simulink model "Model_Compare"  (R2018a)
settings: Solver=FixedStepDiscrete  StartTime=0.0  StopTime=37  FixedStep=Ts  RelTol=1e-3  EnableMultiTasking=on
values from neighbouring files (symbols this model uses):
  alpha_f0 = states(7)    [IS_2impulse.m]    (also in IS_3impulse.m; IS_4impulse.m; InputShaper.m; InputShaper2.m = 0)
  alpha_r0 = states(8)    [IS_2impulse.m]    (also in IS_3impulse.m; IS_4impulse.m; InputShaper.m; InputShaper2.m = 0)
  Bx_ash_f = 11.7    [ISData.m]    (also in SbWdata.m; pacjeka_params.m)
  Bx_ash_r = 11.1    [ISData.m]    (also in SbWdata.m; pacjeka_params.m)
  Bx_snow_f = 10.2    [ISData.m]    (also in SbWdata.m; pacjeka_params.m)
  Bx_snow_r = 9.71    [ISData.m]    (also in SbWdata.m; pacjeka_params.m)
  Bx_wash_f = 12    [ISData.m]    (also in SbWdata.m; pacjeka_params.m)
  Bx_wash_r = 11.5    [ISData.m]    (also in SbWdata.m; pacjeka_params.m)
  By_ash_f = 8.86    [ISData.m]    (also in SbWdata.m; pacjeka_params.m)
  By_ash_r = 9.30    (= 9.3)    [ISData.m]    (also in SbWdata.m; pacjeka_params.m)
  By_snow_f = 19.1    [ISData.m]    (also in SbWdata.m; pacjeka_params.m)
  By_snow_r = 20.0    (= 20)    [ISData.m]    (also in SbWdata.m; pacjeka_params.m)
  By_wash_f = 10.7    [ISData.m]    (also in SbWdata.m; pacjeka_params.m)
  By_wash_r = 11.3    [ISData.m]    (also in SbWdata.m; pacjeka_params.m)
  Cx_ash_f = 1.69    [ISData.m]    (also in SbWdata.m; pacjeka_params.m)
  Cx_ash_r = 1.69    [ISData.m]    (also in SbWdata.m; pacjeka_params.m)
  Cx_snow_f = 1.96    [ISData.m]    (also in SbWdata.m; pacjeka_params.m)
  Cx_snow_r = 1.96    [ISData.m]    (also in SbWdata.m; pacjeka_params.m)
  Cx_wash_f = 1.80    (= 1.8)    [ISData.m]    (also in SbWdata.m; pacjeka_params.m)
  Cx_wash_r = 1.80    (= 1.8)    [ISData.m]    (also in SbWdata.m; pacjeka_params.m)
  Cy_ash_f = 1.19    [ISData.m]    (also in SbWdata.m; pacjeka_params.m)
  Cy_ash_r = 1.19    [ISData.m]    (also in SbWdata.m; pacjeka_params.m)
  Cy_snow_f = 0.550    (= 0.55)    [ISData.m]    (also in SbWdata.m; pacjeka_params.m)
  Cy_snow_r = 0.550    (= 0.55)    [ISData.m]    (also in SbWdata.m; pacjeka_params.m)
  Cy_wash_f = 1.07    [ISData.m]    (also in SbWdata.m; pacjeka_params.m)
  Cy_wash_r = 1.07    [ISData.m]    (also in SbWdata.m; pacjeka_params.m)
  D_phi = 16000    [ISData.m]    (also in IS_2impulse.m; IS_3impulse.m; IS_4impulse.m; InputShaper.m)
  D_theta = 30960    [ISData.m]    (also in IS_2impulse.m; IS_3impulse.m; IS_4impulse.m; InputShaper.m)
  delta_r = 0    [ISData.m]    (also in IS_2impulse.m; IS_3impulse.m; IS_4impulse.m; InputShaper.m)
  epsilon = 0.4    [ISData.m]    (also in IS_2impulse.m; IS_3impulse.m; IS_4impulse.m; InputShaper.m)
  Ex_ash_f = 0.377    [ISData.m]    (also in SbWdata.m; pacjeka_params.m)
  Ex_ash_r = 0.362    [ISData.m]    (also in SbWdata.m; pacjeka_params.m)
  Ex_snow_f = 0.651    [ISData.m]    (also in SbWdata.m; pacjeka_params.m)
  Ex_snow_r = 0.624    [ISData.m]    (also in SbWdata.m; pacjeka_params.m)
  Ex_wash_f = 0.313    [ISData.m]    (also in SbWdata.m; pacjeka_params.m)
  Ex_wash_r = 0.300    (= 0.3)    [ISData.m]    (also in SbWdata.m; pacjeka_params.m)
  Ey_ash_f = -1.21    [ISData.m]    (also in SbWdata.m; pacjeka_params.m)
  Ey_ash_r = -1.11    [ISData.m]    (also in SbWdata.m; pacjeka_params.m)
  Ey_snow_f = -2.1    [ISData.m]    (also in SbWdata.m; pacjeka_params.m)
  Ey_snow_r = -1.93    [ISData.m]    (also in SbWdata.m; pacjeka_params.m)
  Ey_wash_f = -2.14    [ISData.m]    (also in SbWdata.m; pacjeka_params.m)
  Ey_wash_r = -1.97    [ISData.m]    (also in SbWdata.m; pacjeka_params.m)
  g = 9.81    [ISData.m]    (also in IS_2impulse.m; IS_3impulse.m; IS_4impulse.m; InputShaper.m)
  h = 0.5    [ISData.m]    (also in IS_2impulse.m; IS_3impulse.m; IS_4impulse.m; InputShaper.m)
  Iw = 4    [ISData.m]    (also in IS_2impulse.m; IS_3impulse.m; IS_4impulse.m; InputShaper.m)
  Ixx = 602.1923    [ISData.m]    (also in IS_2impulse.m; IS_3impulse.m; IS_4impulse.m; InputShaper.m)
  Iyy = 2.7370e+03    (= 2737)    [ISData.m]    (also in IS_2impulse.m; IS_3impulse.m; IS_4impulse.m; InputShaper.m)
  Iz = Izz    (= 3070)    [IS_2impulse.m]    (also in IS_3impulse.m; IS_4impulse.m; InputShaper.m; InputShaper2.m)
  Izz = 3070    [ISData.m]    (also in IS_2impulse.m; IS_3impulse.m; IS_4impulse.m; InputShaper.m)
  K_phi = 178000    [ISData.m]    (also in IS_2impulse.m; IS_3impulse.m; IS_4impulse.m; InputShaper.m)
  K_theta = 363540    [ISData.m]    (also in IS_2impulse.m; IS_3impulse.m; IS_4impulse.m; InputShaper.m)
  l = l_f+l_r    (= 2.67)    [IS_2impulse.m]    (also in IS_3impulse.m; IS_4impulse.m; InputShaper.m; InputShaper2.m)
  l_f = 1.2110    (= 1.211)    [ISData.m]    (also in IS_2impulse.m; IS_3impulse.m; IS_4impulse.m; InputShaper.m)
  l_r = 1.4590    (= 1.459)    [ISData.m]    (also in IS_2impulse.m; IS_3impulse.m; IS_4impulse.m; InputShaper.m)
  m = 1830    [ISData.m]    (also in IS_2impulse.m; IS_3impulse.m; IS_4impulse.m; InputShaper.m)
  mu_x_ash_f = 1.20    (= 1.2)    [ISData.m]    (also in SbWdata.m; pacjeka_params.m)
  mu_x_ash_r = 1.20    (= 1.2)    [ISData.m]    (also in SbWdata.m; pacjeka_params.m)
  mu_x_snow_f = 0.407    [ISData.m]    (also in SbWdata.m; pacjeka_params.m)
  mu_x_snow_r = 0.409    [ISData.m]    (also in SbWdata.m; pacjeka_params.m)
  mu_x_wash_f = 1.06    [ISData.m]    (also in SbWdata.m; pacjeka_params.m)
  mu_x_wash_r = 1.07    [ISData.m]    (also in SbWdata.m; pacjeka_params.m)
  mu_y_ash_f = 0.935    [ISData.m]    (also in SbWdata.m; pacjeka_params.m)
  mu_y_ash_r = 0.961    [ISData.m]    (also in SbWdata.m; pacjeka_params.m)
  mu_y_snow_f = 0.383    [ISData.m]    (also in SbWdata.m; pacjeka_params.m)
  mu_y_snow_r = 0.394    [ISData.m]    (also in SbWdata.m; pacjeka_params.m)
  mu_y_wash_f = 0.885    [ISData.m]    (also in SbWdata.m; pacjeka_params.m)
  mu_y_wash_r = 0.911    [ISData.m]    (also in SbWdata.m; pacjeka_params.m)
  omega0 = Vx0/Rw    (= 48.6005830904)    [ISData.m]    (also in IS_2impulse.m = 74.1; IS_3impulse.m = 74.1; IS_4impulse.m = 74.1; InputShaper.m = 55.5666666667)
  omega_f0 = states(5)    [IS_2impulse.m]    (also in IS_3impulse.m; IS_4impulse.m; InputShaper.m; InputShaper2.m = 55.5666666667)
  omega_r0 = states(6)    [IS_2impulse.m]    (also in IS_3impulse.m; IS_4impulse.m; InputShaper.m; InputShaper2.m = 55.5666666667)
  psi0 = states(2)    [IS_2impulse.m]    (also in IS_3impulse.m; IS_4impulse.m; InputShaper.m; InputShaper2.m = 0)
  psi_dot0 = states(1)    [IS_2impulse.m]    (also in IS_3impulse.m; IS_4impulse.m; InputShaper.m; InputShaper2.m = 0)
  Px0 = states(9)    [IS_2impulse.m]    (also in IS_3impulse.m; IS_4impulse.m; InputShaper.m; InputShaper2.m = 0)
  Py0 = states(10)    [IS_2impulse.m]    (also in IS_3impulse.m; IS_4impulse.m; InputShaper.m; InputShaper2.m = 0)
  Re = Rw    (= 0.3)    [IS_2impulse.m]    (also in IS_3impulse.m; IS_4impulse.m; InputShaper.m; InputShaper2.m)
  road = 1    [ISData.m]    (also in IS_2impulse.m; IS_3impulse.m; IS_4impulse.m; InputShaper.m)
  Rw = 0.3430    (= 0.343)    [ISData.m]    (also in IS_2impulse.m = 0.3; IS_3impulse.m = 0.3; IS_4impulse.m = 0.3; InputShaper.m = 0.3)
  sigma = epsilon    (= 0.4)    [IS_2impulse.m]    (also in IS_3impulse.m; IS_4impulse.m; InputShaper.m; InputShaper2.m)
  Ts = 0.001    [ISData.m]    (also in IS_2impulse.m; IS_3impulse.m; IS_4impulse.m; InputShaper.m)
  Tsmall = 0.001    [ISData.m]    (also in IS_2impulse.m; IS_3impulse.m; IS_4impulse.m; InputShaper.m)
  Vx0 = 16.67    [ISData.m]    (also in IS_2impulse.m = states(3); IS_3impulse.m = states(3); IS_4impulse.m = states(3); InputShaper.m = states(3))
  Vy0 = states(4)    [IS_2impulse.m]    (also in IS_3impulse.m; IS_4impulse.m; InputShaper.m; InputShaper2.m = 0)
  w = 0.7700    (= 0.77)    [ISData.m]    (also in IS_2impulse.m; IS_3impulse.m; IS_4impulse.m; InputShaper.m)
undefined symbols (not defined in the file or in its folder): theta_sw_FH
libraries: simulink x2
(part 1 of 3)
settings Model: ExtModeTrigDuration=10000  Creator=srivats  LastModifiedBy=srivats
settings SolverCC: PositivePriorityOrder=on
settings RTWCC: SystemTargetFile=quarc_win64.tlc  TemplateMakefile=quarc_default_tmf  Description=QUARC Win64 Target
settings STFCustomTargetCC: TargetPreCompLibLocation=C:\PROGRA~3\QUARC\lib\2018a\win64\release  TargetLangStandard=C99 (ISO)  ConcurrentExecutionCompliant=on  SystemTargetFile=quarc_win64.tlc
settings GRTTargetCC: TargetPreCompLibLocation=C:\PROGRA~3\QUARC\lib\2018a\win64\release  ParMdlRefBuildCompliant=off  CompOptLevelCompliant=off  CombineOutputUpdateFcns=off  MatFileLogging=off  CPPClassGenCompliant=off  GRTInterface=on  UseToolchainInfoCompliant=off  ExtMode=on  ExtModeMexFile=quarc_comm

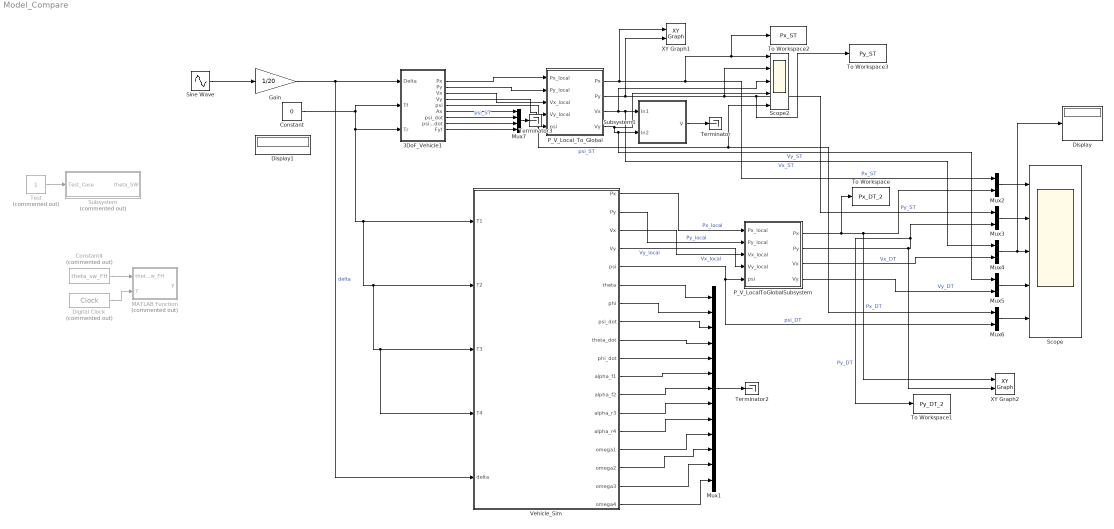
== system Model_Compare ==
  3DoF_Vehicle1 : Subsystem
  Constant : Constant  Value=0
  Constant4 : Constant  Commented=on  Value=theta_sw_FH
  Digital Clock : DigitalClock  Commented=on  SampleTime=0.001
  Display : Display
  Display1 : Display
  Gain : Gain  Gain=1/20
  MATLAB Function : MATLAB Function  Commented=on  TreatAsAtomicUnit=on
  Mux1 : Mux  Inputs=13
  Mux{2..6} (5 alike) : Mux  Inputs=2
  Mux7 : Mux
  P_V_LocalToGlobalSubsystem : Subsystem
  P_V_Local_To_Global : Subsystem
  Scope : Scope  NumInputPorts=5
  Scope2 : Scope  NumInputPorts=5
  Sine Wave : Sin  Amplitude=0.11  Frequency=2*pi/10  SampleTime=0
  Subsystem : Subsystem  Commented=on
  Subsystem1 : Subsystem
  Terminator : Terminator
  Terminator2 : Terminator
  Terminator3 : Terminator
  Test : Constant  Commented=on
  To Workspace : ToWorkspace  VariableName=Px_DT_2  SaveFormat=Timeseries  SampleTime=-1
  To Workspace1 : ToWorkspace  VariableName=Py_DT_2  SaveFormat=Timeseries  SampleTime=-1
  To Workspace2 : ToWorkspace  VariableName=Px_ST  SaveFormat=Timeseries  SampleTime=-1
  To Workspace3 : ToWorkspace  VariableName=Py_ST  SaveFormat=Timeseries  SampleTime=-1
  Vehicle_Sim : Subsystem
  XY Graph1 : simulink/Sinks/XY Graph  xmin=0  xmax=1000  ymin=-100  ymax=100  st=-1
  XY Graph2 : simulink/Sinks/XY Graph  xmin=0  xmax=1000  ymin=-100  ymax=100  st=-1
  wires:
  3DoF_Vehicle1/7(psi_dot) -> Mux7/2  "psi_ST"
  Subsystem1/1(V) -> Terminator/1
  3DoF_Vehicle1/3(Vx) -> P_V_Local_To_Global/3(Vx_local)
  3DoF_Vehicle1/1(Px) -> P_V_Local_To_Global/1(Px_local)
  3DoF_Vehicle1/4(Vy) -> P_V_Local_To_Global/4(Vy_local)
  3DoF_Vehicle1/2(Py) -> P_V_Local_To_Global/2(Py_local)
  P_V_Local_To_Global/4(Vy) -> Scope2/4, Mux5/1, Subsystem1/2(In2)  "Vy_ST"
  P_V_Local_To_Global/3(Vx) -> Scope2/3, Mux4/1, Subsystem1/1(In1)  "Vx_ST"
  Gain/1 -> Vehicle_Sim/5("delta "), 3DoF_Vehicle1/1(Delta)  "delta"
  P_V_LocalToGlobalSubsystem/4(Vy) -> Mux5/2  "Vy_DT"
  Vehicle_Sim/6(theta) -> Mux1/1
  Vehicle_Sim/7(phi) -> Mux1/2
  Vehicle_Sim/17(omega3) -> Mux1/12
  Vehicle_Sim/2(Py) -> P_V_LocalToGlobalSubsystem/2(Py_local)  "Py_local"
  Vehicle_Sim/18(omega4) -> Mux1/13
  Vehicle_Sim/11(alpha_f1) -> Mux1/6
  P_V_LocalToGlobalSubsystem/2(Py) -> XY Graph2/2, To Workspace1/1, Mux3/2  "Py_DT"
  P_V_LocalToGlobalSubsystem/3(Vx) -> Mux4/2  "Vx_DT"
  P_V_LocalToGlobalSubsystem/1(Px) -> To Workspace/1, XY Graph2/1, Mux2/2  "Px_DT"
  Vehicle_Sim/8(psi_dot) -> Mux1/3
  Vehicle_Sim/4(Vy) -> P_V_LocalToGlobalSubsystem/4(Vy_local)  "Vy_local"
  Mux1/1 -> Terminator2/1
  Vehicle_Sim/1(Px) -> P_V_LocalToGlobalSubsystem/1(Px_local)  "Px_local"
  Vehicle_Sim/12(alpha_f2) -> Mux1/7
  Vehicle_Sim/10(phi_dot) -> Mux1/5
  Vehicle_Sim/3(Vx) -> P_V_LocalToGlobalSubsystem/3(Vx_local)  "Vx_local"
  Vehicle_Sim/14(alpha_r4) -> Mux1/9
  Vehicle_Sim/15(omega1) -> Mux1/10
  Vehicle_Sim/5(psi) -> Mux6/2, P_V_LocalToGlobalSubsystem/5(psi)  "psi_DT"
  Vehicle_Sim/16(omega2) -> Mux1/11
  Vehicle_Sim/9(theta_dot) -> Mux1/4
  Vehicle_Sim/13(alpha_r3) -> Mux1/8
  P_V_Local_To_Global/1(Px) -> XY Graph1/1, To Workspace2/1, Scope2/1, Mux2/1  "Px_ST"
  Mux2/1 -> Scope/1
  P_V_Local_To_Global/2(Py) -> XY Graph1/2, Scope2/2, To Workspace3/1, Mux3/1  "Py_ST"
  Mux3/1 -> Scope/2
  Mux4/1 -> Display/1, Scope/3
  Mux5/1 -> Scope/4
  Mux6/1 -> Scope/5
  Constant/1 -> Vehicle_Sim/4(T4), Vehicle_Sim/3(T3), Vehicle_Sim/2(T2), Vehicle_Sim/1(T1), 3DoF_Vehicle1/3(Tr), 3DoF_Vehicle1/2(Tf)
  3DoF_Vehicle1/6(Ax) -> Mux7/1
  3DoF_Vehicle1/8(psi_ddot) -> Mux7/3
  3DoF_Vehicle1/9(Fyf) -> Mux7/4
  Mux7/1 -> Terminator3/1
  3DoF_Vehicle1/5(psi) -> Scope2/5, Mux6/1, P_V_Local_To_Global/5(psi)  "psi_ST"
  Test/1 -> Subsystem/1(Test_Case)
  Digital Clock/1 -> MATLAB Function/2(T)
  Constant4/1 -> MATLAB Function/1(theta_sw_FH)
  Sine Wave/1 -> Gain/1

== system Model_Compare/3DoF_Vehicle1 ==
  Delta : Inport
  Tf : Inport  Port=2
  Tr : Inport  Port=3
  Add : Sum
  Add1 : Sum
  Add2 : Sum
  Constant : Constant  Value=Px0
  Constant1 : Constant  Value=Py0
  Constant2 : Constant  Value=psi0
  Constant3 : Constant  Value=psi_dot0
  Constant4 : Constant  Value=Vy0
  Constant5 : Constant  Value=Vx0
  Constant6 : Constant  Value=omega_f0
  Constant7 : Constant  Value=omega_r0
  Constant8 : Constant  Value=alpha_f0
  Constant9 : Constant  Value=alpha_r0
  Delay : Delay  DelayLength=1  InitialConditionSource=Input port  SampleTime=Tsmall
      settings: InputPortMap=u0,p4
  Delay1 : Delay  DelayLength=1  InitialConditionSource=Input port  SampleTime=Tsmall
      settings: InputPortMap=u0,p4
  Demux : Demux  Outputs=8
  Demux1 : Demux  Outputs=2
  Gain : Gain  Gain=Tsmall
  Gain1 : Gain  Gain=Tsmall
  Gain2 : Gain  Gain=Tsmall
  Mux : Mux  Inputs=8
  Mux1 : Mux  Inputs=2
  Mux2 : Mux  Inputs=2
  Mux3 : Mux  Inputs=8
  Subsystem1 : Subsystem
  Px : Outport
  Py : Outport  Port=2
  Vx : Outport  Port=3
  Vy : Outport  Port=4
  psi : Outport  Port=5
  Ax : Outport  Port=6
  psi_dot : Outport  Port=7
  psi_ddot : Outport  Port=8
  Fyf : Outport  Port=9
  wires:
  Demux/1 -> psi/1, Add/2  "psi_curr"
  Delay/1 -> Demux/1
  Demux/6 -> Subsystem1/6(omega_r_curr)  "omega_r_curr"
  Gain/1 -> Add/1
  Delta/1 -> Subsystem1/1(Delta)
  Subsystem1/4(omega_f_next) -> Mux/5  "omega_f_next"
  Subsystem1/1(psi_dot_next) -> Mux/2, Gain/1  "psi_dot_next"
  Add/1 -> Mux/1  "psi_next"
  Tr/1 -> Subsystem1/8(Tr)
  Tf/1 -> Subsystem1/7(Tf)
  Subsystem1/3(Vx_next) -> Mux/4  "Vx_next"
  Demux/2 -> psi_dot/1, Subsystem1/2(psi_dot_curr)  "psi_dot_curr"
  Mux/1 -> Delay/1
  Demux/4 -> Vx/1, Gain1/1, Subsystem1/3(Vx_curr)  "Vx_curr"
  Demux/3 -> Gain2/1, Subsystem1/4(Vy_curr), Vy/1  "Vy_curr"
  Demux/5 -> Subsystem1/5(omega_f_curr)  "omega_f_curr"
  Subsystem1/2(Vy_next) -> Mux/3  "Vy_next"
  Subsystem1/5(omega_r_next) -> Mux/6  "omega_r_next"
  Gain1/1 -> Add1/1
  Gain2/1 -> Add2/1
  Mux1/1 -> Delay1/1
  Add1/1 -> Mux1/1  "Px_next"
  Add2/1 -> Mux1/2  "Py_next"
  Mux2/1 -> Delay1/2
  Constant/1 -> Mux2/1
  Constant1/1 -> Mux2/2
  Delay1/1 -> Demux1/1
  Demux1/1 -> Add1/2, Px/1  "Px_curr"
  Demux1/2 -> Add2/2, Py/1  "Py_curr"
  Constant7/1 -> Mux3/6
  Constant6/1 -> Mux3/5
  Constant3/1 -> Mux3/2
  Constant5/1 -> Mux3/4
  Constant4/1 -> Mux3/3
  Constant2/1 -> Mux3/1
  Mux3/1 -> Delay/2
  Subsystem1/6(alpha_f_next) -> Mux/7  "alpha_f_next"
  Subsystem1/7(alpha_r_next) -> Mux/8  "alpha_r_next"
  Constant8/1 -> Mux3/7
  Constant9/1 -> Mux3/8
  Demux/7 -> Subsystem1/9(alpha_f_curr)  "alpha_f_curr"
  Demux/8 -> Subsystem1/10(alpha_r_curr)  "alpha_r_curr"
  Subsystem1/8(Ax) -> Ax/1
  Subsystem1/9(psi_ddot) -> psi_ddot/1
  Subsystem1/10(Fyf) -> Fyf/1

== system Model_Compare/P_V_LocalToGlobalSubsystem ==
  Px_local : Inport  OutDataTypeStr=double  SampleTime=Ts
  Py_local : Inport  Port=2  OutDataTypeStr=double  SampleTime=Ts
  Vx_local : Inport  Port=3  OutDataTypeStr=double  SampleTime=Ts
  Vy_local : Inport  Port=4  OutDataTypeStr=double  SampleTime=Ts
  psi : Inport  Port=5  OutDataTypeStr=double  SampleTime=Ts
  Add : Sum  Inputs=+-
  Add1 : Sum
  Add2 : Sum  Inputs=+-
  Add3 : Sum
  Cos : Trigonometry  Operator=cos
  Product{,1..7} (8 alike) : Product
  Sin : Trigonometry
  Px : Outport  OutDataTypeStr=double  SampleTime=Ts
  Py : Outport  Port=2  OutDataTypeStr=double  SampleTime=Ts
  Vx : Outport  Port=3  OutDataTypeStr=double  SampleTime=Ts
  Vy : Outport  Port=4  OutDataTypeStr=double  SampleTime=Ts
  wires:
  Px_local/1 -> Product6/1, Product4/1  "Px_local"
  Py_local/1 -> Product7/1, Product5/1  "Py_local"
  Vx_local/1 -> Product2/1, Product/2  "Vx_local"
  Product5/1 -> Add2/2
  Product4/1 -> Add2/1
  Add2/1 -> Px/1  "Px"
  Product7/1 -> Add3/2
  Vy_local/1 -> Product3/1, Product1/2  "Vy_local"
  psi/1 -> Sin/1, Cos/1  "psi"
  Cos/1 -> Product3/2, Product/1, Product7/2, Product4/2  "cosPsi"
  Add3/1 -> Py/1  "Py"
  Product2/1 -> Add1/1
  Product1/1 -> Add/2
  Add/1 -> Vx/1  "Vx"
  Add1/1 -> Vy/1  "Vy"
  Product6/1 -> Add3/1
  Product3/1 -> Add1/2
  Product/1 -> Add/1
  Sin/1 -> Product2/2, Product1/1, Product6/2, Product5/2  "sinPsi"

== system Model_Compare/P_V_Local_To_Global ==
  Px_local : Inport  OutDataTypeStr=double  SampleTime=Ts
  Py_local : Inport  Port=2  OutDataTypeStr=double  SampleTime=Ts
  Vx_local : Inport  Port=3  OutDataTypeStr=double  SampleTime=Ts
  Vy_local : Inport  Port=4  OutDataTypeStr=double  SampleTime=Ts
  psi : Inport  Port=5  OutDataTypeStr=double  SampleTime=Ts
  Add : Sum  Inputs=+-
  Add1 : Sum
  Add2 : Sum  Inputs=+-
  Add3 : Sum
  Cos : Trigonometry  Operator=cos
  Product{,1..7} (8 alike) : Product
  Sin : Trigonometry
  Px : Outport  OutDataTypeStr=double  SampleTime=Ts
  Py : Outport  Port=2  OutDataTypeStr=double  SampleTime=Ts
  Vx : Outport  Port=3  OutDataTypeStr=double  SampleTime=Ts
  Vy : Outport  Port=4  OutDataTypeStr=double  SampleTime=Ts
  wires:
  Px_local/1 -> Product4/1, Product6/2
  Py_local/1 -> Product7/1, Product5/1
  Vx_local/1 -> Product3/1, Product/1
  Product5/1 -> Add2/2
  Product4/1 -> Add2/1
  Add2/1 -> Px/1  "Px"
  Product7/1 -> Add3/2
  Sin/1 -> Product6/1, Product5/2, Product3/2, Product1/1  "sinPsi"
  Vy_local/1 -> Product1/2, Product2/2
  psi/1 -> Sin/1, Cos/1
  Cos/1 -> Product7/2, Product4/2, Product2/1, Product/2  "cosPsi"
  Add3/1 -> Py/1  "Py"
  Product2/1 -> Add1/1
  Product1/1 -> Add/2
  Add/1 -> Vx/1  "Vx"
  Add1/1 -> Vy/1  "Vy"
  Product6/1 -> Add3/1
  Product3/1 -> Add1/2
  Product/1 -> Add/1

== system Model_Compare/Subsystem ==
  Test_Case : Inport
  If : If  IfExpression=u1==1  ElseIfExpressions=u1==2  ShowElse=off
  If Action Subsystem : Subsystem  TreatAsAtomicUnit=on
  If Action Subsystem1 : Subsystem  TreatAsAtomicUnit=on
  Merge : Merge
  theta_SW : Outport
  wires:
  Merge/1 -> theta_SW/1
  Test_Case/1 -> If/1
  If Action Subsystem/1(Out1) -> Merge/1
  If/1 -> If Action Subsystem/Action
  If/2 -> If Action Subsystem1/Action
  If Action Subsystem1/1(Out1) -> Merge/2

== system Model_Compare/Subsystem1 ==
  In1 : Inport
  In2 : Inport  Port=2
  Add : Sum
  Sqrt : Sqrt  SaturateOnIntegerOverflow=on
  Square : Math  Operator=square  SaturateOnIntegerOverflow=on
  Square1 : Math  Operator=square  SaturateOnIntegerOverflow=on
  V : Outport
  wires:
  Square1/1 -> Add/2
  In1/1 -> Square/1
  Add/1 -> Sqrt/1
  Square/1 -> Add/1
  Sqrt/1 -> V/1  "V"
  In2/1 -> Square1/1

== system Model_Compare/Vehicle_Sim ==
  T1 : Inport  OutDataTypeStr=double  SampleTime=Ts
  T2 : Inport  Port=2  OutDataTypeStr=double  SampleTime=Ts
  T3 : Inport  Port=3  OutDataTypeStr=double  SampleTime=Ts
  T4 : Inport  Port=4  OutDataTypeStr=double  SampleTime=Ts
  "delta " : Inport  Port=5
  Add1 : Sum
  Add2 : Sum
  Delay2 : Delay  DelayLength=1  SampleTime=Tsmall
  Delay3 : Delay  DelayLength=1  SampleTime=Tsmall
  Demux : Demux  Outputs=11
  Demux1 : Demux
  Gain1 : Gain  Gain=Tsmall
  Gain2 : Gain  Gain=Tsmall
  Mux : Mux  Inputs=11
      settings: DisplayOption=signals
  Mux1 : Mux
      settings: DisplayOption=signals
  Vehicle_model : Subsystem
  Vx_delay : Delay  DelayLength=1  InitialCondition=Vx0  SampleTime=Tsmall
  omega_delay : Delay  DelayLength=1  InitialCondition=omega0*ones(4,1)  SampleTime=Tsmall
  otherstates_delay : Delay  DelayLength=1  InitialCondition=zeros(11,1)  SampleTime=Tsmall
  Px : Outport  OutDataTypeStr=double  SampleTime=Tsmall
  Py : Outport  Port=2  OutDataTypeStr=double  SampleTime=Tsmall
  Vx : Outport  Port=3  OutDataTypeStr=double  SampleTime=Tsmall
  Vy : Outport  Port=4  OutDataTypeStr=double  SampleTime=Tsmall
  psi : Outport  Port=5  OutDataTypeStr=double  SampleTime=Tsmall
  theta : Outport  Port=6  OutDataTypeStr=double  SampleTime=Tsmall
  phi : Outport  Port=7  OutDataTypeStr=double  SampleTime=Tsmall
  psi_dot : Outport  Port=8  OutDataTypeStr=double  SampleTime=Tsmall
  theta_dot : Outport  Port=9  OutDataTypeStr=double  SampleTime=Tsmall
  phi_dot : Outport  Port=10  OutDataTypeStr=double  SampleTime=Tsmall
  alpha_f1 : Outport  Port=11  OutDataTypeStr=double  SampleTime=Tsmall
  alpha_f2 : Outport  Port=12  OutDataTypeStr=double  SampleTime=Tsmall
  alpha_r3 : Outport  Port=13  OutDataTypeStr=double  SampleTime=Tsmall
  alpha_r4 : Outport  Port=14  OutDataTypeStr=double  SampleTime=Tsmall
  omega1 : Outport  Port=15  OutDataTypeStr=double  SampleTime=Tsmall
  omega2 : Outport  Port=16  OutDataTypeStr=double  SampleTime=Tsmall
  omega3 : Outport  Port=17  OutDataTypeStr=double  SampleTime=Tsmall
  omega4 : Outport  Port=18  OutDataTypeStr=double  SampleTime=Tsmall
  wires:
  Vehicle_model/14(theta_next) -> Mux/9  "theta_next"
  Vehicle_model/12(psi_next) -> Mux/7  "psi_next"
  Vehicle_model/11(psi_dot_next) -> Mux/6  "psi_dot_next"
  Vehicle_model/15(phi_dot_next) -> Mux/10  "phi_dot_next"
  Mux/1 -> otherstates_delay/1
  Vehicle_model/3(alpha_f1_next) -> Mux/2  "alpha_f1_next"
  Vehicle_model/5(alpha_r3_next) -> Mux/4  "alpha_r3_next"
  Vehicle_model/9(omega3_next) -> Mux1/3  "omega3_next"
  Vehicle_model/8(omega2_next) -> Mux1/2  "omega2_next"
  Vehicle_model/13(theta_dot_next) -> Mux/8  "theta_dot_next"
  Vehicle_model/4(alpha_f2_next) -> Mux/3  "alpha_f2_next"
  Vehicle_model/6(alpha_r4_next) -> Mux/5  "alpha_r4_next"
  Vehicle_model/10(omega4_next) -> Mux1/4  "omega4_next"
  Vehicle_model/1(Vx_next) -> Vx_delay/1  "Vx_next"
  Demux/1 -> Gain2/1, Vy/1, Vehicle_model/6(Vy_curr)
  Vehicle_model/7(omega1_next) -> Mux1/1  "omega1_next"
  Demux1/3 -> omega3/1, Vehicle_model/13(omega3_curr)
  Demux/5 -> Vehicle_model/10(alpha_r4_curr), alpha_r4/1
  Demux/8 -> theta_dot/1, Vehicle_model/17(theta_dot_curr)
  Vehicle_model/16(phi_next) -> Mux/11  "phi_next"
  Vehicle_model/2(Vy_next) -> Mux/1  "Vy_next"
  T1/1 -> Vehicle_model/1(T1)
  Add2/1 -> Delay3/1
  Delay3/1 -> Py/1, Add2/2  "Py_curr"
  Add1/1 -> Delay2/1  "Px_next"
  Delay2/1 -> Px/1, Add1/2  "Px_curr"
  Gain1/1 -> Add1/1
  Gain2/1 -> Add2/1
  T3/1 -> Vehicle_model/3(T3)
  T4/1 -> Vehicle_model/4(T4)
  T2/1 -> Vehicle_model/2(T2)
  otherstates_delay/1 -> Demux/1
  Demux/4 -> Vehicle_model/9(alpha_r3_curr), alpha_r3/1
  Demux/11 -> phi/1, Vehicle_model/19(phi_curr)
  Demux/2 -> Vehicle_model/7(alpha_f1_curr), alpha_f1/1
  Demux/3 -> Vehicle_model/8(alpha_f2_curr), alpha_f2/1
  Demux1/4 -> omega4/1, Vehicle_model/14(omega4_curr)
  Demux/7 -> psi/1, Vehicle_model/16(psi_curr)
  Demux/9 -> theta/1, Vehicle_model/18(theta_curr)
  Demux/10 -> phi_dot/1, Vehicle_model/20(phi_dot_curr)
  Demux/6 -> psi_dot/1, Vehicle_model/15(psi_dot_curr)
  Demux1/2 -> omega2/1, Vehicle_model/12(omega2_curr)
  Vx_delay/1 -> Vx/1, Vehicle_model/5(Vx_curr), Gain1/1
  Demux1/1 -> omega1/1, Vehicle_model/11(omega1_curr)
  Mux1/1 -> omega_delay/1
  omega_delay/1 -> Demux1/1
  "delta "/1 -> Vehicle_model/21(delta)

== system Model_Compare/3DoF_Vehicle1/Subsystem1 ==
  Delta : Inport
  psi_dot_curr : Inport  Port=2
  Vx_curr : Inport  Port=3
  Vy_curr : Inport  Port=4
  omega_f_curr : Inport  Port=5
  omega_r_curr : Inport  Port=6
  Tf : Inport  Port=7
  Tr : Inport  Port=8
  alpha_f_curr : Inport  Port=9
  alpha_r_curr : Inport  Port=10
  Cos : Trigonometry  Operator=cos
  Demux1 : Demux  Outputs=8
  Demux2 : Demux  Outputs=8
  Fx_Fy_Subsystem : Subsystem
  Fz_Subsystem : Subsystem
  Omega_k_alpha_Subsystem : Subsystem
  Pacjeka_parameters_Subsystem : Subsystem
  Psi_ddot_subsystem : Subsystem
  Sin : Trigonometry
  Vxdot_subsystem : Subsystem
  Vydot_subsystem : Subsystem
  surface : Constant  Value=road
  psi_dot_next : Outport
  Vy_next : Outport  Port=2
  Vx_next : Outport  Port=3
  omega_f_next : Outport  Port=4
  omega_r_next : Outport  Port=5
  alpha_f_next : Outport  Port=6
  alpha_r_next : Outport  Port=7
  Ax : Outport  Port=8
  psi_ddot : Outport  Port=9
  Fyf : Outport  Port=10
  wires:
  Omega_k_alpha_Subsystem/4(k_r) -> Fx_Fy_Subsystem/21(k_r)
  Fx_Fy_Subsystem/2(Fx_r) -> Vxdot_subsystem/4(Fxr), Omega_k_alpha_Subsystem/10(Fx_r)
  Fx_Fy_Subsystem/1(Fx_f) -> Omega_k_alpha_Subsystem/9(Fx_f), Vxdot_subsystem/3(Fxf), Psi_ddot_subsystem/5(Fxf), Vydot_subsystem/5(Fxf)
  Omega_k_alpha_Subsystem/3(k_f) -> Fx_Fy_Subsystem/22(k_f)
  Sin/1 -> Fx_Fy_Subsystem/24(sinDelta), Vxdot_subsystem/7(sinDelta), Vydot_subsystem/7(sinDelta), Psi_ddot_subsystem/2(sinDelta)
  Vydot_subsystem/1(Vy_next) -> Vy_next/1
  Fx_Fy_Subsystem/3(Fy_f) -> Fyf/1, Psi_ddot_subsystem/3(Fyf), Vydot_subsystem/3(Fyf), Vxdot_subsystem/5(Fyf)
  psi_dot_curr/1 -> Omega_k_alpha_Subsystem/6(psi_dot), Vydot_subsystem/1(psi_dot_curr), Vxdot_subsystem/1(psi_dot_curr), Psi_ddot_subsystem/6(psi_dot_curr)
  Fx_Fy_Subsystem/4(Fy_r) -> Psi_ddot_subsystem/4(Fyr), Vydot_subsystem/4(Fyr)
  Cos/1 -> Fx_Fy_Subsystem/23(cosDelta), Vxdot_subsystem/6(cosDelta), Vydot_subsystem/6(cosDelta), Psi_ddot_subsystem/1(cosDelta)
  Tf/1 -> Omega_k_alpha_Subsystem/7(Tf)
  Demux1/7 -> Fx_Fy_Subsystem/17(E_x_f)  "E_x_f"
  omega_f_curr/1 -> Omega_k_alpha_Subsystem/4(omega_f_curr)
  Vy_curr/1 -> Omega_k_alpha_Subsystem/3(Vy), Vxdot_subsystem/2(Vy_curr), Vydot_subsystem/8(Vy_curr)
  Pacjeka_parameters_Subsystem/1(front) -> Demux1/1
  Omega_k_alpha_Subsystem/6(omega_r_next) -> omega_r_next/1
  Delta/1 -> Omega_k_alpha_Subsystem/1(delta), Sin/1, Cos/1
  Vx_curr/1 -> Omega_k_alpha_Subsystem/2(Vx), Vydot_subsystem/2(Vx_curr), Vxdot_subsystem/8(Vx_curr)
  Demux1/1 -> Fx_Fy_Subsystem/11(mu_x_f)  "mu_x_f"
  Vxdot_subsystem/1(Vx_next) -> Vx_next/1
  Omega_k_alpha_Subsystem/5(omega_f_next) -> omega_f_next/1
  Demux2/4 -> Fx_Fy_Subsystem/6(C_y_r)  "C_y_r"
  Fz_Subsystem/1(Fz_f) -> Fx_Fy_Subsystem/1(Fz_f)
  Tr/1 -> Omega_k_alpha_Subsystem/8(Tr)
  omega_r_curr/1 -> Omega_k_alpha_Subsystem/5(omega_r_curr)
  surface/1 -> Pacjeka_parameters_Subsystem/1(surface_condition)
  Pacjeka_parameters_Subsystem/2(rear) -> Demux2/1
  Demux2/7 -> Fx_Fy_Subsystem/9(E_x_r)  "E_x_r"
  Fz_Subsystem/2(Fz_r) -> Fx_Fy_Subsystem/2(Fz_r)
  Demux1/6 -> Fx_Fy_Subsystem/16(B_y_f)  "B_y_f"
  Demux2/6 -> Fx_Fy_Subsystem/8(B_y_r)  "B_y_r"
  Demux2/2 -> Fx_Fy_Subsystem/4(mu_y_r)  "mu_y_r"
  Demux1/8 -> Fx_Fy_Subsystem/18(E_y_f)  "E_y_f"
  Demux2/5 -> Fx_Fy_Subsystem/7(B_x_r)  "B_x_r"
  Psi_ddot_subsystem/1(psi_dot_next) -> psi_dot_next/1
  Demux2/8 -> Fx_Fy_Subsystem/10(E_y_r)  "E_y_r"
  Demux2/1 -> Fx_Fy_Subsystem/3(mu_x_r)  "mu_x_r"
  Demux1/3 -> Fx_Fy_Subsystem/13(C_x_f)  "C_x_f"
  Demux1/4 -> Fx_Fy_Subsystem/14(C_y_f)  "C_y_f"
  Demux1/2 -> Fx_Fy_Subsystem/12(mu_y_f)  "mu_y_f"
  Demux1/5 -> Fx_Fy_Subsystem/15(B_x_f)  "B_x_f"
  Demux2/3 -> Fx_Fy_Subsystem/5(C_x_r)  "C_x_r"
  Omega_k_alpha_Subsystem/1(alpha_f_next) -> alpha_f_next/1
  Omega_k_alpha_Subsystem/2(alpha_r_next) -> alpha_r_next/1
  alpha_r_curr/1 -> Fx_Fy_Subsystem/20(alpha_r), Omega_k_alpha_Subsystem/12(alpha_r_curr)
  alpha_f_curr/1 -> Fx_Fy_Subsystem/19(alpha_f), Omega_k_alpha_Subsystem/11(alpha_f_curr)
  Vxdot_subsystem/2(Ax) -> Ax/1
  Psi_ddot_subsystem/2(psi_ddot) -> psi_ddot/1

== system Model_Compare/Subsystem/If Action Subsystem ==
  Action Port : ActionPort  ActionType=then
  From Workspace : FromWorkspace  VariableName=theta_SW_FH  SampleTime=0
  Out1 : Outport
  wires:
  From Workspace/1 -> Out1/1

== system Model_Compare/Subsystem/If Action Subsystem1 ==
  Action Port : ActionPort  ActionType=elseif
  Constant : Constant  Value=0
  Out1 : Outport
  wires:
  Constant/1 -> Out1/1

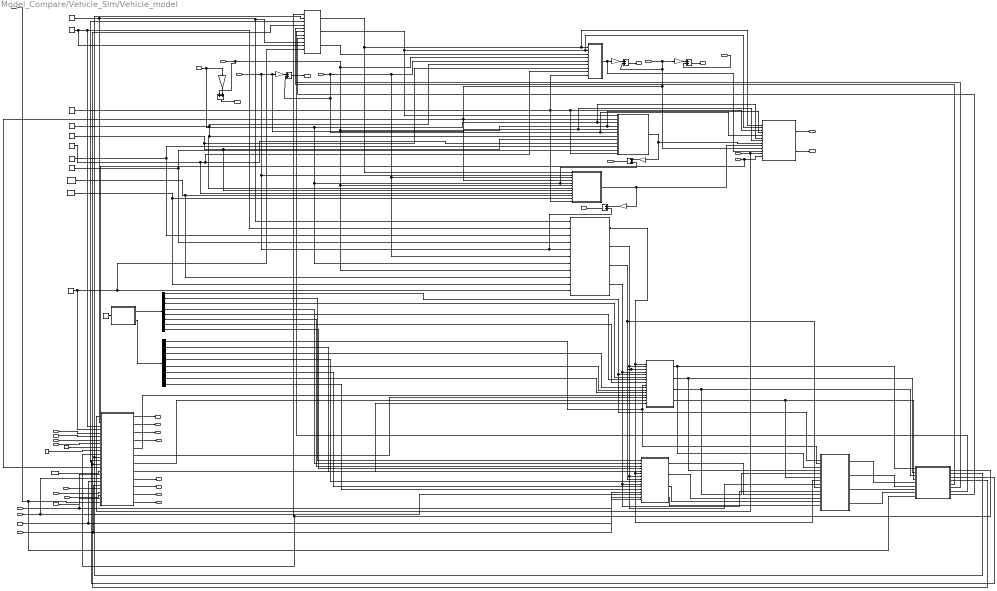
== system Model_Compare/Vehicle_Sim/Vehicle_model ==
  T1 : Inport  OutDataTypeStr=double  SampleTime=Ts
  T2 : Inport  Port=2  OutDataTypeStr=double  SampleTime=Ts
  T3 : Inport  Port=3  OutDataTypeStr=double  SampleTime=Ts
  T4 : Inport  Port=4  OutDataTypeStr=double  SampleTime=Ts
  Vx_curr : Inport  Port=5  OutDataTypeStr=double  SampleTime=Tsmall
  Vy_curr : Inport  Port=6  OutDataTypeStr=double  SampleTime=Tsmall
  alpha_f1_curr : Inport  Port=7  OutDataTypeStr=double  SampleTime=Tsmall
  alpha_f2_curr : Inport  Port=8  OutDataTypeStr=double  SampleTime=Tsmall
  alpha_r3_curr : Inport  Port=9  OutDataTypeStr=double  SampleTime=Tsmall
  alpha_r4_curr : Inport  Port=10  OutDataTypeStr=double  SampleTime=Tsmall
  omega1_curr : Inport  Port=11  OutDataTypeStr=double  SampleTime=Tsmall
  omega2_curr : Inport  Port=12  OutDataTypeStr=double  SampleTime=Tsmall
  omega3_curr : Inport  Port=13  OutDataTypeStr=double  SampleTime=Tsmall
  omega4_curr : Inport  Port=14  OutDataTypeStr=double  SampleTime=Tsmall
  psi_dot_curr : Inport  Port=15  OutDataTypeStr=double  SampleTime=Tsmall
  psi_curr : Inport  Port=16  OutDataTypeStr=double  SampleTime=Tsmall
  theta_dot_curr : Inport  Port=17  OutDataTypeStr=double  SampleTime=Tsmall
  theta_curr : Inport  Port=18  OutDataTypeStr=double  SampleTime=Tsmall
  phi_curr : Inport  Port=19  OutDataTypeStr=double  SampleTime=Tsmall
  phi_dot_curr : Inport  Port=20  OutDataTypeStr=double  SampleTime=Tsmall
  delta : Inport  Port=21  OutDataTypeStr=double  SampleTime=Tsmall
  Add{,1..5} (6 alike) : Sum
  D_phi : Constant  Value=D_phi
  D_theta : Constant  Value=D_theta
  Demux1 : Demux  Outputs=8
  Demux2 : Demux  Outputs=8
  F_M_subsystem : Subsystem
  Fx0_Subsystem : Subsystem
  Fy0_Subsystem : Subsystem
  Fy0_to_Fy_subsystem : Subsystem
  Fz_Subsystem : Subsystem
  Gain{,1..5} (6 alike) : Gain  Gain=Tsmall
  Iw : Constant  Value=Iw
  Ixx : Constant  Value=Ixx
  Iyy : Constant  Value=Iyy
  Izz : Constant  Value=Izz
  K_phi : Constant  Value=K_phi
  K_theta : Constant  Value=K_theta
  Pacjeka_parameters_Subsystem : Subsystem
  Rw : Constant  Value=Rw
  Vx_Vy_Subsystem : Subsystem
  epsilon : Constant  Value=epsilon
  h : Constant  Value=h
  l_f : Constant  Value=l_f
  l_r : Constant  Value=l_r
  local_to_global_Fx_Fy_Subsystem : Subsystem
  omega_alpha_and_k_values_subsystem : Subsystem
  phi_subsystem : Subsystem
  psi_subsystem : Subsystem
  surface : Constant  Value=road
  theta_subsystem : Subsystem
  w : Constant  Value=w
  Vx_next : Outport  OutDataTypeStr=double  SampleTime=Tsmall
  Vy_next : Outport  Port=2  OutDataTypeStr=double  SampleTime=Tsmall
  alpha_f1_next : Outport  Port=3  OutDataTypeStr=double  SampleTime=Tsmall
  alpha_f2_next : Outport  Port=4  OutDataTypeStr=double  SampleTime=Tsmall
  alpha_r3_next : Outport  Port=5  OutDataTypeStr=double  SampleTime=Tsmall
  alpha_r4_next : Outport  Port=6  OutDataTypeStr=double  SampleTime=Tsmall
  omega1_next : Outport  Port=7  OutDataTypeStr=double  SampleTime=Tsmall
  omega2_next : Outport  Port=8  OutDataTypeStr=double  SampleTime=Tsmall
  omega3_next : Outport  Port=9  OutDataTypeStr=double  SampleTime=Tsmall
  omega4_next : Outport  Port=10  OutDataTypeStr=double  SampleTime=Tsmall
  psi_dot_next : Outport  Port=11  OutDataTypeStr=double  SampleTime=Tsmall
  psi_next : Outport  Port=12  OutDataTypeStr=double  SampleTime=Tsmall
  theta_dot_next : Outport  Port=13  OutDataTypeStr=double  SampleTime=Tsmall
  theta_next : Outport  Port=14  OutDataTypeStr=double  SampleTime=Tsmall
  phi_dot_next : Outport  Port=15  OutDataTypeStr=double  SampleTime=Tsmall
  phi_next : Outport  Port=16  OutDataTypeStr=double  SampleTime=Tsmall
  wires:
  Add/1 -> psi_dot_next/1
  Gain4/1 -> Add4/1
  Gain5/1 -> Add5/2
  Add4/1 -> phi_dot_next/1
  Add5/1 -> phi_next/1
  omega1_curr/1 -> omega_alpha_and_k_values_subsystem/22(omega1_curr)
  omega3_curr/1 -> omega_alpha_and_k_values_subsystem/24(omega3_curr)
  omega_alpha_and_k_values_subsystem/11(omega3_next) -> omega3_next/1
  omega_alpha_and_k_values_subsystem/12(omega4_next) -> omega4_next/1
  F_M_subsystem/2(FY) -> phi_subsystem/1(FY), Vx_Vy_Subsystem/2(FY), psi_subsystem/2(FY)  "Fy"
  theta_curr/1 -> Add3/2, Vx_Vy_Subsystem/5(theta), phi_subsystem/6(theta), psi_subsystem/5(theta), Fz_Subsystem/6(theta), theta_subsystem/3(theta)
  Ixx/1 -> psi_subsystem/6(Ixx), theta_subsystem/7(Ixx), phi_subsystem/7(Ixx)  "Ixx"
  phi_dot_curr/1 -> Vx_Vy_Subsystem/6(phi_dot), phi_subsystem/3(phi_dot), Add4/2, theta_subsystem/5(phi_dot), Fz_Subsystem/7(phi_dot), Gain5/1  "phi_dot"
  Izz/1 -> theta_subsystem/9(Izz), psi_subsystem/8(Izz), phi_subsystem/9(Izz)  "Izz"
  theta_subsystem/1(theta_ddot) -> Vx_Vy_Subsystem/9(theta_ddot), Gain2/1  "theta_ddot"
  K_phi/1 -> Fz_Subsystem/3(k_phi), phi_subsystem/10(K_phi)  "k_phi"
  F_M_subsystem/1(FX) -> theta_subsystem/1(FX), Vx_Vy_Subsystem/1(FX), psi_subsystem/1(FX)  "Fx"
  phi_curr/1 -> Add5/1, Fz_Subsystem/8(phi), theta_subsystem/6(phi), Vx_Vy_Subsystem/4(phi), phi_subsystem/4(phi), psi_subsystem/4(phi)
  theta_dot_curr/1 -> Gain3/1, Vx_Vy_Subsystem/7(theta_dot), phi_subsystem/5(theta_dot), theta_subsystem/2(theta_dot), Add2/2, Fz_Subsystem/5(theta_dot)
  F_M_subsystem/3(Mz) -> psi_subsystem/3(MZ)  "MZ"
  psi_subsystem/1(psi_ddot) -> Gain/1, Vx_Vy_Subsystem/11(psi_ddot)  "psi_ddot"
  phi_subsystem/1(phi_ddot) -> Vx_Vy_Subsystem/8(phi_ddot), Gain4/1  "phi_ddot"
  Iyy/1 -> psi_subsystem/7(Iyy), theta_subsystem/8(Iyy), phi_subsystem/8(Iyy)  "Iyy"
  D_theta/1 -> Fz_Subsystem/10(D_theta), theta_subsystem/11(D_theta)  "D_theta"
  Pacjeka_parameters_Subsystem/1(front) -> Demux1/1
  w/1 -> omega_alpha_and_k_values_subsystem/5(w), F_M_subsystem/11(w), Fz_Subsystem/11(w)  "w"
  Demux1/4 -> Fy0_Subsystem/2(C_y_f)  "C_y_f"
  Demux1/2 -> Fy0_Subsystem/1(mu_y_f)  "mu_y_f"
  Fz_Subsystem/2(Fz2) -> Fy0_to_Fy_subsystem/8(Fz2), Fy0_Subsystem/7(Fz2), Fx0_Subsystem/2(Fz2)  "Fz2"
  Demux2/1 -> Fy0_to_Fy_subsystem/2(mu_x_r), Fx0_Subsystem/9(mu_x_r)  "mu_x_r"
  omega_alpha_and_k_values_subsystem/6(k_f2) -> Fx0_Subsystem/14(k_f2)  "k_f2"
  Demux1/8 -> Fy0_Subsystem/4(E_y_f)  "E_y_f"
  Demux1/6 -> Fy0_Subsystem/3(B_y_f)  "B_y_f"
  surface/1 -> Pacjeka_parameters_Subsystem/1(surface_condition)
  l_r/1 -> F_M_subsystem/10(l_r), omega_alpha_and_k_values_subsystem/4(l_r), Fz_Subsystem/2(l_r)  "l_r"
  Fz_Subsystem/4(Fz4) -> Fy0_to_Fy_subsystem/10(Fz4), Fy0_Subsystem/10(Fz4), Fx0_Subsystem/4(Fz4)  "Fz4"
  Demux1/5 -> Fx0_Subsystem/7(B_x_f)  "B_x_f"
  Demux1/7 -> Fx0_Subsystem/8(E_x_f)  "E_x_f"
  D_phi/1 -> Fz_Subsystem/4(d_phi), phi_subsystem/11(D_phi)  "d_phi"
  omega_alpha_and_k_values_subsystem/5(k_f1) -> Fx0_Subsystem/13(k_f1)  "k_f1"
  Demux1/1 -> Fy0_to_Fy_subsystem/1(mu_x_f), Fx0_Subsystem/5(mu_x_f)  "mu_x_f"
  omega_alpha_and_k_values_subsystem/7(k_r3) -> Fx0_Subsystem/15(k_r3)  "k_r3"
  l_f/1 -> omega_alpha_and_k_values_subsystem/3(l_f), F_M_subsystem/9(l_f), Fz_Subsystem/1(l_f)  "l_f"
  K_theta/1 -> Fz_Subsystem/9(K_theta), theta_subsystem/10(K_theta)  "K_theta"
  Demux2/3 -> Fx0_Subsystem/10(C_x_r)  "C_x_r"
  Demux2/7 -> Fx0_Subsystem/12(E_x_r)  "E_x_r"
  Pacjeka_parameters_Subsystem/2(rear) -> Demux2/1
  omega_alpha_and_k_values_subsystem/8(k_r4) -> Fx0_Subsystem/16(k_r4)  "k_r4"
  Fx0_Subsystem/1(Fx01) -> local_to_global_Fx_Fy_Subsystem/1(local_Fx1), Fy0_to_Fy_subsystem/3(Fx01)  "Fx01"
  Demux1/3 -> Fx0_Subsystem/6(C_x_f)  "C_x_f"
  Demux2/5 -> Fx0_Subsystem/11(B_x_r)  "B_x_r"
  Fz_Subsystem/1(Fz1) -> Fx0_Subsystem/1(Fz1), Fy0_to_Fy_subsystem/7(Fz1), Fy0_Subsystem/6(Fz1)  "Fz1"
  Demux2/6 -> Fy0_Subsystem/11(B_y_r)  "B_y_r"
  Fz_Subsystem/3(Fz3) -> Fy0_to_Fy_subsystem/9(Fz3), Fx0_Subsystem/3(Fz3), Fy0_Subsystem/8(Fz3)  "Fz3"
  local_to_global_Fx_Fy_Subsystem/6(Fy2) -> F_M_subsystem/6(Fy2)  "Fy2"
  T4/1 -> omega_alpha_and_k_values_subsystem/9(T4)
  Demux2/8 -> Fy0_Subsystem/12(E_y_r)  "E_y_r"
  Fy0_Subsystem/4(Fy04) -> Fy0_to_Fy_subsystem/14(Fy04)  "Fy04"
  alpha_f1_curr/1 -> omega_alpha_and_k_values_subsystem/18(alpha_f1_curr), Fy0_Subsystem/13(alpha_f1)
  epsilon/1 -> omega_alpha_and_k_values_subsystem/17(epsilon)
  Vx_Vy_Subsystem/1(Vx_next) -> Vx_next/1
  Fx0_Subsystem/4(Fx04) -> local_to_global_Fx_Fy_Subsystem/4(local_Fx4), Fy0_to_Fy_subsystem/6(Fx04)  "Fx04"
  alpha_f2_curr/1 -> Fy0_Subsystem/14(alpha_f2), omega_alpha_and_k_values_subsystem/19(alpha_f2_curr)
  Fy0_Subsystem/1(Fy01) -> Fy0_to_Fy_subsystem/11(Fy01)  "Fy01"
  Fy0_Subsystem/2(Fy02) -> Fy0_to_Fy_subsystem/12(Fy02)  "Fy02"
  Demux2/4 -> Fy0_Subsystem/9(C_y_r)  "C_y_r"
  local_to_global_Fx_Fy_Subsystem/5(Fy1) -> F_M_subsystem/5(Fy1)  "Fy1"
  Fx0_Subsystem/3(Fx03) -> Fy0_to_Fy_subsystem/5(Fx03), local_to_global_Fx_Fy_Subsystem/3(local_Fx3)  "Fx03"
  local_to_global_Fx_Fy_Subsystem/7(Fy3) -> F_M_subsystem/7(Fy3)  "Fy3"
  Rw/1 -> omega_alpha_and_k_values_subsystem/10(Rw)
  h/1 -> Vx_Vy_Subsystem/3(h), phi_subsystem/12(h), psi_subsystem/9(h), theta_subsystem/12(h)  "h"
  Fx0_Subsystem/2(Fx02) -> local_to_global_Fx_Fy_Subsystem/2(local_Fx2), Fy0_to_Fy_subsystem/4(Fx02)
  local_to_global_Fx_Fy_Subsystem/8(Fy4) -> F_M_subsystem/8(Fy4)  "Fy4"
  T3/1 -> omega_alpha_and_k_values_subsystem/8(T3)
  T1/1 -> omega_alpha_and_k_values_subsystem/6(T1)
  Iw/1 -> omega_alpha_and_k_values_subsystem/11(Iw)
  T2/1 -> omega_alpha_and_k_values_subsystem/7(T2)
  alpha_r4_curr/1 -> Fy0_Subsystem/16(alpha_r4), omega_alpha_and_k_values_subsystem/21(alpha_r4_curr)
  Fy0_Subsystem/3(Fy03) -> Fy0_to_Fy_subsystem/13(Fy03)  "Fy03"
  Demux2/2 -> Fy0_Subsystem/5(mu_y_r)  "mu_y_r"
  alpha_r3_curr/1 -> Fy0_Subsystem/15(alpha_r3), omega_alpha_and_k_values_subsystem/20(alpha_r3_curr)
  Vy_curr/1 -> omega_alpha_and_k_values_subsystem/2(Vy), Vx_Vy_Subsystem/13(Vy_curr)
  omega_alpha_and_k_values_subsystem/3(alpha_r3_next) -> alpha_r3_next/1
  Vx_curr/1 -> omega_alpha_and_k_values_subsystem/1(Vx), Vx_Vy_Subsystem/12(Vx_curr)
  omega_alpha_and_k_values_subsystem/1(alpha_f1_next) -> alpha_f1_next/1  "alpha_f1"
  omega_alpha_and_k_values_subsystem/4(alpha_r4_next) -> alpha_r4_next/1  "alpha_r4"
  Vx_Vy_Subsystem/2(Vy_next) -> Vy_next/1
  omega_alpha_and_k_values_subsystem/2(alpha_f2_next) -> alpha_f2_next/1  "alpha_f2"
  psi_dot_curr/1 -> Gain1/1, Add/2, Vx_Vy_Subsystem/10(psi_dot), omega_alpha_and_k_values_subsystem/16(psi_dot), theta_subsystem/4(psi_dot), phi_subsystem/2(psi_dot)  "psi_dot"
  Gain1/1 -> Add1/1
  psi_curr/1 -> Add1/2
  omega4_curr/1 -> omega_alpha_and_k_values_subsystem/25(omega4_curr)
  omega_alpha_and_k_values_subsystem/10(omega2_next) -> omega2_next/1
  omega2_curr/1 -> omega_alpha_and_k_values_subsystem/23(omega2_curr)
  Gain3/1 -> Add3/1
  Gain2/1 -> Add2/1
  Gain/1 -> Add/1
  Add3/1 -> theta_next/1
  Add2/1 -> theta_dot_next/1
  Add1/1 -> psi_next/1
  omega_alpha_and_k_values_subsystem/9(omega1_next) -> omega1_next/1
  delta/1 -> local_to_global_Fx_Fy_Subsystem/9(delta_f2), omega_alpha_and_k_values_subsystem/26(delta_f2)  "delta_f2"
  Fy0_to_Fy_subsystem/1(local_Fy1) -> local_to_global_Fx_Fy_Subsystem/5(local_Fy1)  "Fy1"
  Fy0_to_Fy_subsystem/2(local_Fy2) -> local_to_global_Fx_Fy_Subsystem/6(local_Fy2)  "Fy2"
  Fy0_to_Fy_subsystem/3(local_Fy3) -> local_to_global_Fx_Fy_Subsystem/7(local_Fy3)  "Fy3"
  Fy0_to_Fy_subsystem/4(lcoal_Fy4) -> local_to_global_Fx_Fy_Subsystem/8(local_Fy4)  "Fy4"
  local_to_global_Fx_Fy_Subsystem/1(Fx1) -> omega_alpha_and_k_values_subsystem/12(Fx1), F_M_subsystem/1(Fx1)  "Fx1"
  local_to_global_Fx_Fy_Subsystem/2(Fx2) -> omega_alpha_and_k_values_subsystem/13(Fx2), F_M_subsystem/2(Fx2)  "Fx2"
  local_to_global_Fx_Fy_Subsystem/3(Fx3) -> F_M_subsystem/3(Fx3), omega_alpha_and_k_values_subsystem/14(Fx3)  "Fx3"
  local_to_global_Fx_Fy_Subsystem/4(Fx4) -> F_M_subsystem/4(Fx4), omega_alpha_and_k_values_subsystem/15(Fx4)  "Fx4"

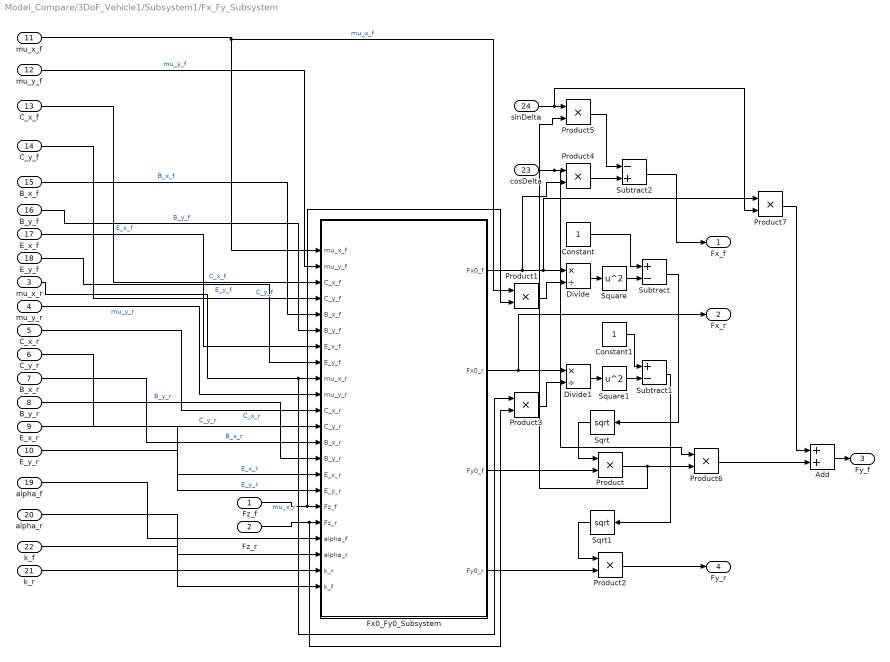
== system Model_Compare/3DoF_Vehicle1/Subsystem1/Fx_Fy_Subsystem ==
  Fz_f : Inport
  Fz_r : Inport  Port=2
  mu_x_r : Inport  Port=3
  mu_y_r : Inport  Port=4
  C_x_r : Inport  Port=5
  C_y_r : Inport  Port=6
  B_x_r : Inport  Port=7
  B_y_r : Inport  Port=8
  E_x_r : Inport  Port=9
  E_y_r : Inport  Port=10
  mu_x_f : Inport  Port=11
  mu_y_f : Inport  Port=12
  C_x_f : Inport  Port=13
  C_y_f : Inport  Port=14
  B_x_f : Inport  Port=15
  B_y_f : Inport  Port=16
  E_x_f : Inport  Port=17
  E_y_f : Inport  Port=18
  alpha_f : Inport  Port=19
  alpha_r : Inport  Port=20
  k_r : Inport  Port=21
  k_f : Inport  Port=22
  cosDelta : Inport  Port=23
  sinDelta : Inport  Port=24
  Add : Sum
  Constant : Constant
  Constant1 : Constant
  Divide : Product  Inputs=*/
  Divide1 : Product  Inputs=*/
  Fx0_Fy0_Subsystem : Subsystem
  Product{,1..7} (8 alike) : Product
  Sqrt : Sqrt  SaturateOnIntegerOverflow=on
  Sqrt1 : Sqrt  SaturateOnIntegerOverflow=on
  Square : Math  Operator=square  SaturateOnIntegerOverflow=on
  Square1 : Math  Operator=square  SaturateOnIntegerOverflow=on
  Subtract : Sum  Inputs=+-
  Subtract1 : Sum  Inputs=+-
  Subtract2 : Sum  Inputs=-+
  Fx_f : Outport
  Fx_r : Outport  Port=2
  Fy_f : Outport  Port=3
  Fy_r : Outport  Port=4
  wires:
  B_x_r/1 -> Fx0_Fy0_Subsystem/13(B_x_r)  "B_x_r"
  mu_y_r/1 -> Fx0_Fy0_Subsystem/10(mu_y_r)  "mu_y_r"
  C_x_r/1 -> Fx0_Fy0_Subsystem/11(C_x_r)  "C_x_r"
  E_y_r/1 -> Fx0_Fy0_Subsystem/16(E_y_r)  "E_y_r"
  mu_x_r/1 -> Fx0_Fy0_Subsystem/9(mu_x_r), Product3/1  "mu_x_r"
  C_y_r/1 -> Fx0_Fy0_Subsystem/12(C_y_r)  "C_y_r"
  E_x_r/1 -> Fx0_Fy0_Subsystem/15(E_x_r)  "E_x_r"
  B_y_r/1 -> Fx0_Fy0_Subsystem/14(B_y_r)  "B_y_r"
  B_x_f/1 -> Fx0_Fy0_Subsystem/5(B_x_f)  "B_x_f"
  mu_y_f/1 -> Fx0_Fy0_Subsystem/2(mu_y_f)  "mu_y_f"
  C_x_f/1 -> Fx0_Fy0_Subsystem/3(C_x_f)  "C_x_f"
  E_y_f/1 -> Fx0_Fy0_Subsystem/8(E_y_f)  "E_y_f"
  mu_x_f/1 -> Product1/1, Fx0_Fy0_Subsystem/1(mu_x_f)  "mu_x_f"
  C_y_f/1 -> Fx0_Fy0_Subsystem/4(C_y_f)  "C_y_f"
  E_x_f/1 -> Fx0_Fy0_Subsystem/7(E_x_f)  "E_x_f"
  B_y_f/1 -> Fx0_Fy0_Subsystem/6(B_y_f)  "B_y_f"
  Fz_f/1 -> Product1/2, Fx0_Fy0_Subsystem/17(Fz_f)
  Fz_r/1 -> Product3/2, Fx0_Fy0_Subsystem/18(Fz_r)
  alpha_f/1 -> Fx0_Fy0_Subsystem/19(alpha_f)
  alpha_r/1 -> Fx0_Fy0_Subsystem/20(alpha_r)
  k_f/1 -> Fx0_Fy0_Subsystem/22(k_f)
  k_r/1 -> Fx0_Fy0_Subsystem/21(k_r)
  Constant/1 -> Subtract/1
  Fx0_Fy0_Subsystem/1(Fx0_f) -> Product4/2, Product7/1, Divide/1
  Product1/1 -> Divide/2
  Divide/1 -> Square/1
  Subtract/1 -> Sqrt/1
  Square/1 -> Subtract/2
  Sqrt/1 -> Product/1
  Product/1 -> Product6/2, Product5/2
  Product2/1 -> Fy_r/1
  Fx0_Fy0_Subsystem/4(Fy0_r) -> Product2/2
  Sqrt1/1 -> Product2/1
  Divide1/1 -> Square1/1
  Square1/1 -> Subtract1/2
  Product3/1 -> Divide1/2
  Fx0_Fy0_Subsystem/2(Fx0_r) -> Fx_r/1, Divide1/1
  Constant1/1 -> Subtract1/1
  Subtract1/1 -> Sqrt1/1
  cosDelta/1 -> Product6/1, Product4/1
  Product4/1 -> Subtract2/2
  sinDelta/1 -> Product7/2, Product5/1
  Fx0_Fy0_Subsystem/3(Fy0_f) -> Product/2
  Product5/1 -> Subtract2/1
  Subtract2/1 -> Fx_f/1
  Product7/1 -> Add/1
  Product6/1 -> Add/2
  Add/1 -> Fy_f/1

== system Model_Compare/3DoF_Vehicle1/Subsystem1/Fz_Subsystem ==
  Constant : Constant  Value=(m*g*l_f)/l
  Constant1 : Constant  Value=(m*g*l_r)/l
  Fz_f : Outport
  Fz_r : Outport  Port=2
  wires:
  Constant/1 -> Fz_r/1
  Constant1/1 -> Fz_f/1

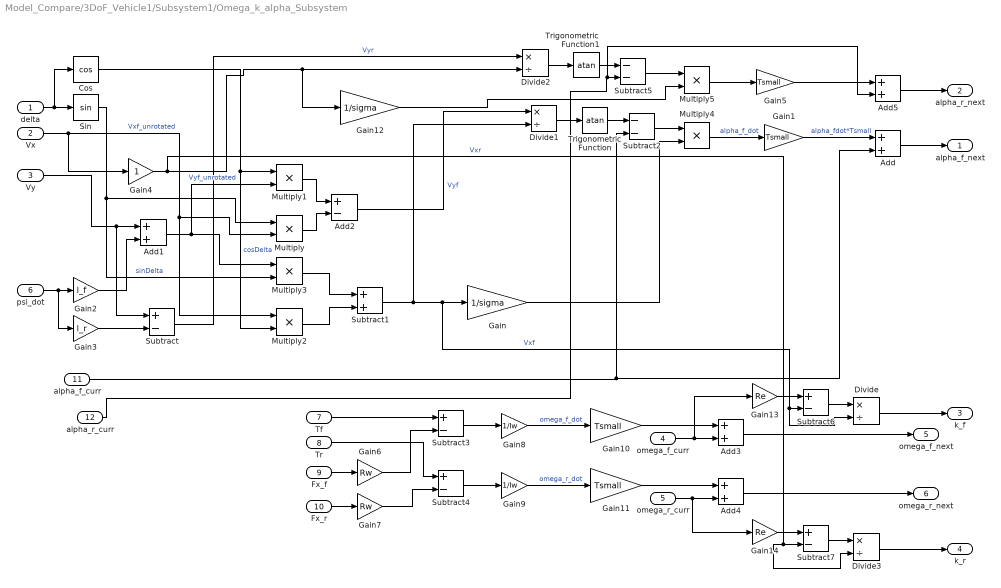
== system Model_Compare/3DoF_Vehicle1/Subsystem1/Omega_k_alpha_Subsystem ==
  delta : Inport
  Vx : Inport  Port=2
  Vy : Inport  Port=3
  omega_f_curr : Inport  Port=4
  omega_r_curr : Inport  Port=5
  psi_dot : Inport  Port=6
  Tf : Inport  Port=7
  Tr : Inport  Port=8
  Fx_f : Inport  Port=9
  Fx_r : Inport  Port=10
  alpha_f_curr : Inport  Port=11
  alpha_r_curr : Inport  Port=12
  Add{,1,3..5} (5 alike) : Sum
  Add2 : Sum  Inputs=+-
  Cos : Trigonometry  Operator=cos
  Divide{,1..3} (4 alike) : Product  Inputs=*/
  Gain : Gain  Gain=1/sigma
  Gain{1,5,10..11} (4 alike) : Gain  Gain=Tsmall
  Gain12 : Gain  Gain=1/sigma
  Gain13 : Gain  Gain=Re
  Gain14 : Gain  Gain=Re
  Gain2 : Gain  Gain=l_f
  Gain3 : Gain  Gain=l_r
  Gain4 : Gain
  Gain6 : Gain  Gain=Rw
  Gain7 : Gain  Gain=Rw
  Gain8 : Gain  Gain=1/Iw
  Gain9 : Gain  Gain=1/Iw
  Multiply{,1..5} (6 alike) : Product
  Sin : Trigonometry
  Subtract{,3..4,6..7} (5 alike) : Sum  Inputs=+-
  Subtract1 : Sum
  Subtract2 : Sum  Inputs=--
  Subtract5 : Sum  Inputs=--
  Trigonometric Function : Trigonometry  Operator=atan
  Trigonometric Function1 : Trigonometry  Operator=atan
  alpha_f_next : Outport
  alpha_r_next : Outport  Port=2
  k_f : Outport  Port=3
  k_r : Outport  Port=4
  omega_f_next : Outport  Port=5
  omega_r_next : Outport  Port=6
  wires:
  Fx_f/1 -> Gain6/1
  Fx_r/1 -> Gain7/1
  Tf/1 -> Subtract3/1
  Gain6/1 -> Subtract3/2
  Tr/1 -> Subtract4/1
  Gain7/1 -> Subtract4/2
  Subtract3/1 -> Gain8/1
  Subtract4/1 -> Gain9/1
  Gain8/1 -> Gain10/1  "omega_f_dot"
  Gain9/1 -> Gain11/1  "omega_r_dot"
  Gain10/1 -> Add3/1
  Gain11/1 -> Add4/1
  Add3/1 -> omega_f_next/1
  Add4/1 -> omega_r_next/1
  omega_f_curr/1 -> Gain13/1, Add3/2
  Multiply4/1 -> Gain1/1  "alpha_f_dot"
  Gain1/1 -> Add/1  "alpha_fdot*Tsmall"
  Divide1/1 -> Trigonometric Function/1
  omega_r_curr/1 -> Gain14/1, Add4/2
  psi_dot/1 -> Gain3/1, Gain2/1
  Gain2/1 -> Add1/2
  Vy/1 -> Subtract/1, Add1/1
  Add1/1 -> Multiply1/2, Multiply3/1  "Vyf_unrotated"
  Gain3/1 -> Subtract/2
  Subtract/1 -> Divide2/1  "Vyr"
  Vx/1 -> Multiply/2, Multiply2/1, Gain4/1  "Vxf_unrotated"
  Gain4/1 -> Subtract7/2, Divide3/2, Gain12/1, Divide2/2  "Vxr"
  delta/1 -> Cos/1, Sin/1
  Cos/1 -> Multiply2/2, Multiply1/1  "cosDelta"
  Multiply1/1 -> Add2/1
  Multiply/1 -> Add2/2
  Add2/1 -> Divide1/1  "Vyf"
  Multiply3/1 -> Subtract1/1
  Multiply2/1 -> Subtract1/2
  Subtract1/1 -> Divide/2, Subtract6/2, Gain/1, Divide1/2  "Vxf"
  Trigonometric Function/1 -> Subtract2/1
  alpha_f_curr/1 -> Add/2, Subtract2/2
  Subtract2/1 -> Multiply4/1
  Gain/1 -> Multiply4/2
  Add/1 -> alpha_f_next/1
  Subtract5/1 -> Multiply5/1
  Trigonometric Function1/1 -> Subtract5/1
  Divide2/1 -> Trigonometric Function1/1
  Multiply5/1 -> Gain5/1
  Gain5/1 -> Add5/1
  Add5/1 -> alpha_r_next/1
  alpha_r_curr/1 -> Add5/2, Subtract5/2
  Gain12/1 -> Multiply5/2
  Gain13/1 -> Subtract6/1
  Subtract6/1 -> Divide/1
  Divide/1 -> k_f/1
  Gain14/1 -> Subtract7/1
  Subtract7/1 -> Divide3/1
  Divide3/1 -> k_r/1
  Sin/1 -> Multiply/1, Multiply3/2  "sinDelta"

== system Model_Compare/3DoF_Vehicle1/Subsystem1/Pacjeka_parameters_Subsystem ==
  surface_condition : Inport  OutDataTypeStr=double  SampleTime=Ts
  Ashphalt_condition_subsystem : Subsystem  TreatAsAtomicUnit=on
  Demux : Demux  Outputs=2
  Ice_condition_subsystem : Subsystem  TreatAsAtomicUnit=on
  Merge : Merge  Inputs=4
  Snow_condition_subsystem : Subsystem  TreatAsAtomicUnit=on
  Switch Case : SwitchCase  CaseConditions={1,2,3,4}  ShowDefaultCase=off
  WetAshphalt_condition_subsystem : Subsystem  TreatAsAtomicUnit=on
  front : Outport  OutDataTypeStr=double  SampleTime=Ts
  rear : Outport  Port=2  OutDataTypeStr=double  SampleTime=Ts
  wires:
  Demux/2 -> rear/1  "rear"
  Merge/1 -> Demux/1
  Switch Case/1 -> Ashphalt_condition_subsystem/Action
  Switch Case/3 -> Snow_condition_subsystem/Action
  Demux/1 -> front/1  "front"
  surface_condition/1 -> Switch Case/1
  Ashphalt_condition_subsystem/1(Out1) -> Merge/1
  Switch Case/2 -> WetAshphalt_condition_subsystem/Action
  WetAshphalt_condition_subsystem/1(Out1) -> Merge/2
  Snow_condition_subsystem/1(Out1) -> Merge/3
  Ice_condition_subsystem/1(Out1) -> Merge/4
  Switch Case/4 -> Ice_condition_subsystem/Action

== system Model_Compare/3DoF_Vehicle1/Subsystem1/Psi_ddot_subsystem ==
  cosDelta : Inport
  sinDelta : Inport  Port=2
  Fyf : Inport  Port=3
  Fyr : Inport  Port=4
  Fxf : Inport  Port=5
  psi_dot_curr : Inport  Port=6
  Add : Sum  Inputs=+-
  Add1 : Sum
  Gain : Gain  Gain=l_f
  Gain1 : Gain  Gain=l_r
  Gain3 : Gain  Gain=1/Iz
  Gain4 : Gain  Gain=Tsmall
  Mux : Mux  Inputs=3
  Terminator : Terminator
  psi_dot_next : Outport
  psi_ddot : Outport  Port=2
  wires:
  Gain/1 -> Add/1
  Gain1/1 -> Add/2
  Add/1 -> Gain3/1  "Mz"
  Gain3/1 -> psi_ddot/1, Gain4/1  "psi_ddot"
  Gain4/1 -> Add1/1
  Add1/1 -> psi_dot_next/1  "psi_dot_next"
  Fyf/1 -> Gain/1
  Fyr/1 -> Gain1/1
  psi_dot_curr/1 -> Add1/2
  cosDelta/1 -> Mux/3
  Fxf/1 -> Mux/1
  sinDelta/1 -> Mux/2
  Mux/1 -> Terminator/1

== system Model_Compare/3DoF_Vehicle1/Subsystem1/Vxdot_subsystem ==
  psi_dot_curr : Inport
  Vy_curr : Inport  Port=2
  Fxf : Inport  Port=3
  Fxr : Inport  Port=4
  Fyf : Inport  Port=5
  cosDelta : Inport  Port=6
  sinDelta : Inport  Port=7
  Vx_curr : Inport  Port=8
  Add : Sum
  Fy_subsystem : Subsystem
  Gain : Gain  Gain=1/m
  Gain1 : Gain  Gain=Ts
  Multiply : Product
  Subtract : Sum
  Vx_next : Outport
  Ax : Outport  Port=2
  wires:
  sinDelta/1 -> Fy_subsystem/5(sinDelta)
  cosDelta/1 -> Fy_subsystem/4(cosDelta)
  Fyf/1 -> Fy_subsystem/3(Fxr)
  Fxr/1 -> Fy_subsystem/2(Fxf)
  Fxf/1 -> Fy_subsystem/1(Fyf)
  Fy_subsystem/1(Fx) -> Gain/1
  Gain/1 -> Subtract/2
  psi_dot_curr/1 -> Multiply/1
  Vy_curr/1 -> Multiply/2
  Multiply/1 -> Subtract/1
  Subtract/1 -> Ax/1, Gain1/1
  Gain1/1 -> Add/1
  Vx_curr/1 -> Add/2
  Add/1 -> Vx_next/1  "Vx_next"

== system Model_Compare/3DoF_Vehicle1/Subsystem1/Vydot_subsystem ==
  psi_dot_curr : Inport
  Vx_curr : Inport  Port=2
  Fyf : Inport  Port=3
  Fyr : Inport  Port=4
  Fxf : Inport  Port=5
  cosDelta : Inport  Port=6
  sinDelta : Inport  Port=7
  Vy_curr : Inport  Port=8
  Add : Sum
  Fy_subsystem : Subsystem
  Gain : Gain  Gain=1/m
  Gain1 : Gain  Gain=Ts
  Multiply : Product
  Subtract : Sum  Inputs=-+
  Vy_next : Outport
  wires:
  sinDelta/1 -> Fy_subsystem/5(sinDelta)
  cosDelta/1 -> Fy_subsystem/4(cosDelta)
  Fxf/1 -> Fy_subsystem/3(Fxf)
  Fyr/1 -> Fy_subsystem/2(Fyr)
  Fyf/1 -> Fy_subsystem/1(Fyf)
  Fy_subsystem/1(Fy) -> Gain/1
  Gain/1 -> Subtract/2
  psi_dot_curr/1 -> Multiply/1
  Vx_curr/1 -> Multiply/2
  Multiply/1 -> Subtract/1
  Subtract/1 -> Gain1/1
  Gain1/1 -> Add/1
  Vy_curr/1 -> Add/2
  Add/1 -> Vy_next/1  "Vy_next"
